simulink model "All_injectors_LQG_bop_plasma_ss_model"  (R2022a)
settings: Solver=FixedStepAuto  StartTime=0.0  StopTime=RunTime  FixedStep=SampleTime  RelTol=1e-3
values from neighbouring files (symbols this model uses):
  K_plasma = dlqr(sys_d_plasma.A, sys_d_plasma.B ,Q_cost_tilde,R_cost, 0)    [All_injectors_LQG_bop_plasma_ss_model_code.m]    (also in All_injectors_LQG_bop_ss_model_code.m = lqr(sys_d_plasma,Q_cost,R_cost); All_injectors_LQG_continuous_time_code.m = lqr(sys_d_plasma,Q_cost,R_cost); All_injectors_LQG_plasma_7_15_24_code.m = lqr(sys_d_plasma,Q_cost,R_cost); All_injectors_LQG_plasma_ss_model_code.m = lqr(sys_d_plasma,Q_cost,R_cost))
  SampleTime = 1e-7    (= 1e-07)    [All_injectors_LQG_bop_plasma_ss_model_code.m]    (also in All_injectors_LQG_bop_ss_model_code.m; All_injectors_LQG_continuous_time_code.m; All_injectors_LQG_plasma_7_15_24_code.m; All_injectors_LQG_plasma_ss_model_code.m)
  sys_d_plasma = c2d(sysc,dT,'zoh')    [All_injectors_LQG_bop_plasma_ss_model_code.m]    (also in All_injectors_LQG_bop_ss_model_code.m; All_injectors_LQG_continuous_time_code.m; All_injectors_LQG_plasma_7_15_24_code.m; All_injectors_LQG_plasma_ss_model_code.m)
  syskf_plasma = ss(Ad-L*Cd, [Bd L], eye(r), 0*[Bd L], dT)    [All_injectors_LQG_bop_plasma_ss_model_code.m]    (also in All_injectors_LQG_bop_ss_model_code.m = ss(Ad-L*Cd, [Bd L], eye(size_A), 0*[Bd L], dT); All_injectors_LQG_continuous_time_code.m = ss(Ad-L*Cd, [Bd L], eye(size_A), 0*[Bd L], dT); All_injectors_LQG_plasma_7_15_24_code.m = ss(Ad-L*Cd, [Bd L], eye(size_A), 0*[Bd L], dT); All_injectors_LQG_plasma_ss_model_code.m = ss(Ad-L*Cd, [Bd L], eye(size_A), 0*[Bd L], dT))
libraries: simulink x1
settings Model: Creator=ducks  LastModifiedBy=ducks
settings DataIOCC: ExternalInput=[t,V]

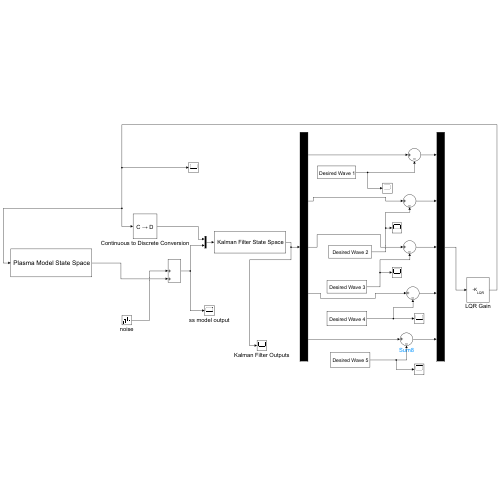
[thumbnail: Simulink's stored preview of the top-level diagram]
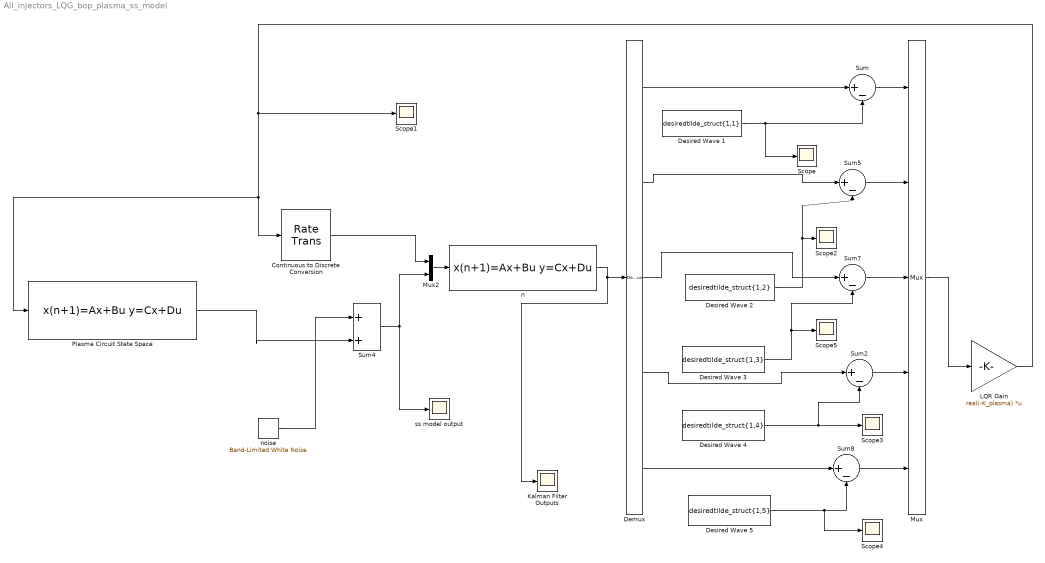
== system All_injectors_LQG_bop_plasma_ss_model ==
  Continuous to Discrete Conversion : RateTransition  OutPortSampleTimeOpt=Inherit
      mask Display: disp('C \rightarrow D','texmode','on');
  Demux : Demux  Outputs=r
  Desired Wave 1 : FromWorkspace  VariableName=desiredtilde_struct{1,1}
      mask Display: disp('\fontsize{16} Desired Wave 1','texmode','on');
  Desired Wave 2 : FromWorkspace  VariableName=desiredtilde_struct{1,2}
      mask Display: disp('\fontsize{16} Desired Wave 2','texmode','on');
  Desired Wave 3 : FromWorkspace  VariableName=desiredtilde_struct{1,3}
      mask Display: disp('\fontsize{16} Desired Wave 3','texmode','on');
  Desired Wave 4 : FromWorkspace  VariableName=desiredtilde_struct{1,4}
      mask Display: disp('\fontsize{16} Desired Wave 4','texmode','on')
  Desired Wave 5 : FromWorkspace  VariableName=desiredtilde_struct{1,5}
      mask Display: disp('\fontsize{16} Desired Wave 5','texmode','on')
  Kalman Filter Outputs : Scope
  LQR Gain : Gain  Gain=real(-K_plasma)  Multiplication=Matrix(K*u) (u vector)
      mask Display: disp('\fontsize{14} -K_{LQR}','texmode','on')
  Mux : Mux  Inputs=r
  Mux2 : Mux  Inputs=2
  Plasma Circuit State Space : DiscreteStateSpace  A=real(sys_d_plasma.A)  B=real(sys_d_plasma.B)  C=real(sys_d_plasma.C)  D=real(sys_d_plasma.D)  SampleTime=-1
      mask Display: disp('\fontsize{20} Plasma Model State Space','texmode','on');
  Scope{,1..5} (6 alike) : Scope
  Sum{,2,5,7..8} (5 alike) : Sum  Inputs=|+-
  Sum4 : Sum  Inputs=|++
  n : DiscreteStateSpace  A=real(syskf_plasma.A)  B=real(syskf_plasma.B)  C=real(syskf_plasma.C)  D=real(syskf_plasma.D)  SampleTime=-1
      mask Display: disp('\fontsize{18} Kalman Filter State Space','texmode','on');
  noise : simulink/Sources/Band-Limited White Noise  Cov=NoisePower  Ts=SampleTime  seed=[23341]
  ss model output : Scope
  wires:
  n/1 -> Kalman Filter Outputs/1, Demux/1
  Plasma Circuit State Space/1 -> Sum4/2
  Continuous to Discrete Conversion/1 -> Mux2/1
  Mux2/1 -> n/1
  noise/1 -> Sum4/1
  Sum4/1 -> Mux2/2, ss model output/1
  Mux/1 -> LQR Gain/1
  LQR Gain/1 -> Scope1/1, Continuous to Discrete Conversion/1, Plasma Circuit State Space/1
  Desired Wave 1/1 -> Scope/1, Sum/2
  Desired Wave 2/1 -> Sum5/2, Scope2/1
  Desired Wave 3/1 -> Sum7/2, Scope5/1
  Desired Wave 5/1 -> Scope4/1, Sum8/2
  Sum2/1 -> Mux/4
  Desired Wave 4/1 -> Sum2/2, Scope3/1
  Demux/4 -> Sum2/1
  Sum7/1 -> Mux/3
  Demux/3 -> Sum7/1
  Demux/2 -> Sum5/1
  Sum/1 -> Mux/1
  Sum5/1 -> Mux/2
  Demux/1 -> Sum/1
  Demux/5 -> Sum8/1
  Sum8/1 -> Mux/5
